simulink subsystem "Control3Leds"  (R2021b)
settings: Solver=VariableStepAuto  StartTime=0.0  StopTime=10.0  RelTol=1e-3
settings Model: Creator=yo  LastModifiedBy=ferna

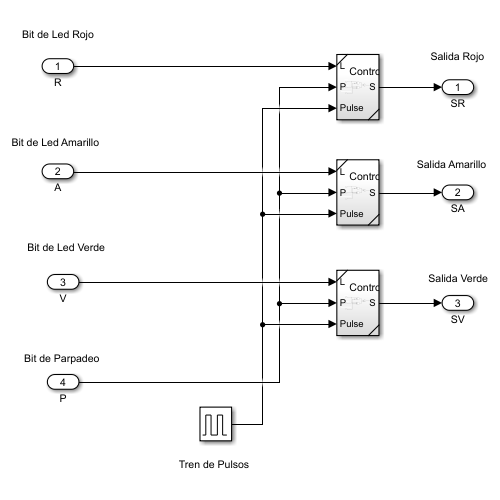
[thumbnail: Simulink's stored preview of the top-level diagram]
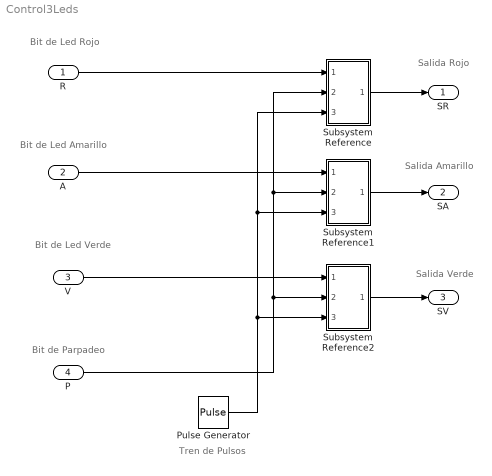
== system Control3Leds ==
  note: Bit de Led Amarillo
  note: Tren de Pulsos
  note: Bit de Led Rojo
  note: Salida Verde
  note: Salida Rojo
  note: Bit de Led Verde
  note: Bit de Parpadeo
  note: Salida Amarillo
  R : Inport
  A : Inport  Port=2
  V : Inport  Port=3
  P : Inport  Port=4
  Pulse Generator : DiscretePulseGenerator  Period=50  PulseWidth=5  SampleTime=0.01
  Subsystem Reference : Subsystem  ReferencedSubsystem=ControlLedUnico
  Subsystem Reference1 : Subsystem  ReferencedSubsystem=ControlLedUnico
  Subsystem Reference2 : Subsystem  ReferencedSubsystem=ControlLedUnico
  SR : Outport
  SA : Outport  Port=2
  SV : Outport  Port=3
  wires:
  Subsystem Reference2/1 -> SV/1
  V/1 -> Subsystem Reference2/1
  P/1 -> Subsystem Reference2/2, Subsystem Reference1/2, Subsystem Reference/2
  Pulse Generator/1 -> Subsystem Reference2/3, Subsystem Reference1/3, Subsystem Reference/3
  Subsystem Reference1/1 -> SA/1
  R/1 -> Subsystem Reference/1
  A/1 -> Subsystem Reference1/1
  Subsystem Reference/1 -> SR/1
